simulink model "bh_filter_test"  (R2026b)
settings: Solver=daessc  StopTime=3  FixedStep=1e-4  MaxStep=0.001  RelTol=1e-5  AbsTol=1e-5  EnableMultiTasking=on
settings Model: Creator=bhorton  LastModifiedBy=bhorton
settings SolverCC: ZeroCrossAlgorithm=Adaptive
settings DataIOCC: LimitDataPoints=on  MaxDataPoints=10000
settings OptimizationCC: LifeSpan=inf  ReuseModelBlockBuffer=off
settings DebuggingCC: AllowSymbolicDim=off  ArithmeticOperatorsInVariantConditions=warning  SFExecutionAtInitializationDiag=none  SFNoUnconditionalDefaultTransitionDiag=warning  SFUnexpectedBacktrackingDiag=warning  SubsystemReferenceDiagnosticForUnitTest=warning
settings SFSimCC: CustomCodeUndefinedFunction=UseInterfaceOnly  SimUseLocalCustomCode=off
settings RTWCC: DLArmComputeVersion=19.05  RTWUseLocalCustomCode=off
settings CodeAppCC: StateflowObjectComments=on
settings GRTTargetCC: TargetLangStandard=C89/C90 (ANSI)
settings ConfigComp: CovExternalEMLEnable=off  CovSFcnEnable=off  CovSaveCumulativeToWorkspaceVar=on  CovSaveSingleToWorkspaceVar=on
settings SimscapeCC: SimscapeLogSimulationStatistics=on  SimscapeLogType=all  SimscapeUseEnergyAccounting=off
settings ExplorerConfigSet: InternalSimMechanicsExplorerSettings="<ExplorerConfiguration><canonicalview>default</canonicalview><TilePanel><TileInfo><Tiles Columns=\"1\" Count=\"1\" Height=\"824\" Rows=\"1\" Width=\"1465\"><Row Weight=\"1\"/><Column Weight=\"1\"/><Tile Height=\"1\" Width=\"1\" X=\"0\" Y=\"0\"/></Tiles></TileInfo><SceneInfo><SceneViewer><IsThisViewStd><IsStandardView>off</IsStandardView><StandardViewName>Front</StandardViewName></IsThisViewStd><BGColor><R>1</R><G>1</G><B>1</B><A>1</A></BGColor><Camera><DoPerspective>off</DoPerspective><Position><X>2.3055029568647205</X><Y>-1.980460360411362</Y><Z>2.4303803604113621</Z></Position><Center><X>0.3250425964533587</X><Y>0</Y><Z>0.44991999999999999</Z></Center><Up><X>-0.40824829046386307</X><Y>0.40824829046386307</Y><Z>0.81649658092772615</Z></Up><XLim>0.56162107958529428</XLim><YLim>0.56162107958529428</YLim><ViewLimDist>0.01</ViewLimDist></Camera></SceneViewer></SceneInfo></TilePanel><MechEditorPanel><GfxPanelCameraMap/><Cameras/><VideoCreator><IncludeTiles>All</IncludeTiles><IncludeTime>on</IncludeTime><IncludeWorldFrame>off</IncludeWorldFrame><PlaybackSpeedRatio>1</PlaybackSpeedRatio><FrameRate>30</FrameRate><FrameSize>auto</FrameSize><VideoFormat>UncompressedAVI</VideoFormat></VideoCreator></MechEditorPanel><PlaybackSettings><PlaybackSpeedFactor>1</PlaybackSpeedFactor></PlaybackSettings></ExplorerConfiguration>"

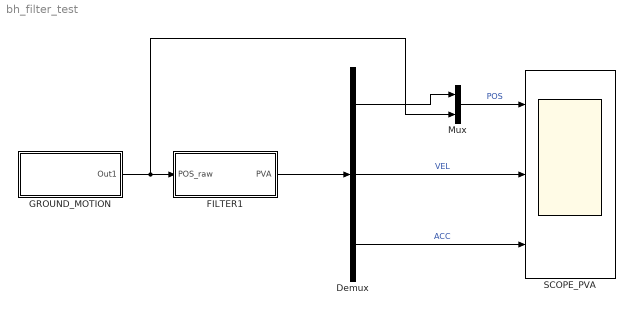
== system bh_filter_test ==
  Demux : Demux  Outputs=3
  FILTER1 : Subsystem  mask(Seconds Order Filter){my_tau=0.01, my_zeta=0.9}
      mask prompts: my_tau "Time constant (seconds)"; my_zeta "Damping RATIO"
      mask help:
      | Smooth input and compute the 1st and 2nd order derivatives of the input.
      |
      | We've parameterised the filter by the time constant TAU and teh damping ratio ZETA
      |   TAU = 1/ (ZETA . w_n )
      |
      | POS = w_n^2  / (s^2    +  2.ZETA.w_n.s   +  w_n^2)
      | VEL  = s . POS
      | ACC = s^2 . POS
      mask init:
      | % w_n = 1/my_tau;
      | 
      | % my_tau = 1 / (w_n * my_zeta)
      | 
      | w_n = (1/my_tau) / my_zeta;
      settings: AttributesFormatString=|
      | Time Constant = %<my_tau>
      | Damp RATIO = %<my_zeta>
      mask DialogControl ParameterGroupVar Prompt: Seconds order filter
  GROUND_MOTION : Subsystem
  Mux : Mux  Inputs=2
  SCOPE_PVA : Scope  NumInputPorts=3
      settings: ActiveDisplayYMinimum=-0.12519495038044745  ActiveDisplayYMaximum=1.1267545534240273
  wires:
  GROUND_MOTION/1(Out1) -> FILTER1/1(POS_raw), Mux/2
  FILTER1/1(PVA) -> Demux/1
  Demux/1 -> Mux/1
  Demux/2 -> SCOPE_PVA/2  "VEL"
  Demux/3 -> SCOPE_PVA/3  "ACC"
  Mux/1 -> SCOPE_PVA/1  "POS"

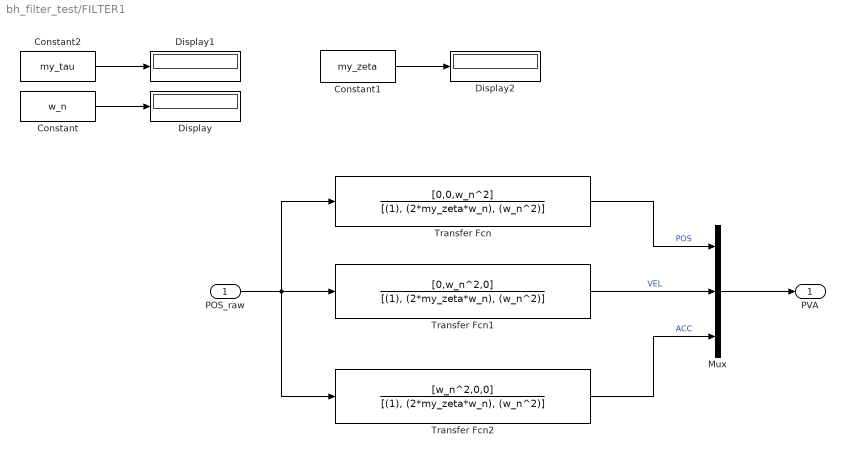
== system bh_filter_test/FILTER1 ==
  POS_raw : Inport
  Constant : Constant  Value=w_n
  Constant1 : Constant  Value=my_zeta
  Constant2 : Constant  Value=my_tau
  Display : Display
  Display1 : Display
  Display2 : Display
  Mux : Mux  Inputs=3
  Transfer Fcn : TransferFcn  Numerator=[0,0,w_n^2]  Denominator=[(1), (2*my_zeta*w_n), (w_n^2)]
  Transfer Fcn1 : TransferFcn  Numerator=[0,w_n^2,0]  Denominator=[(1), (2*my_zeta*w_n), (w_n^2)]
  Transfer Fcn2 : TransferFcn  Numerator=[w_n^2,0,0]  Denominator=[(1), (2*my_zeta*w_n), (w_n^2)]
  PVA : Outport
  wires:
  Constant/1 -> Display/1
  Constant2/1 -> Display1/1
  Constant1/1 -> Display2/1
  POS_raw/1 -> Transfer Fcn/1, Transfer Fcn1/1, Transfer Fcn2/1
  Transfer Fcn/1 -> Mux/1  "POS"
  Transfer Fcn1/1 -> Mux/2  "VEL"
  Transfer Fcn2/1 -> Mux/3  "ACC"
  Mux/1 -> PVA/1

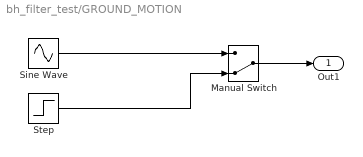
== system bh_filter_test/GROUND_MOTION ==
  Manual Switch : ManualSwitch  CurrentSetting=0
  Sine Wave : Sin  Frequency=2*pi*0.5  SampleTime=0
  Step : Step  SampleTime=0
  Out1 : Outport
  wires:
  Sine Wave/1 -> Manual Switch/1
  Step/1 -> Manual Switch/2
  Manual Switch/1 -> Out1/1
